simulink model "equation"  (R2020b)
settings: Solver=VariableStepAuto  StartTime=0.0  StopTime=10.0  RelTol=1e-3
settings Model: Creator=99003736  LastModifiedBy=99003736

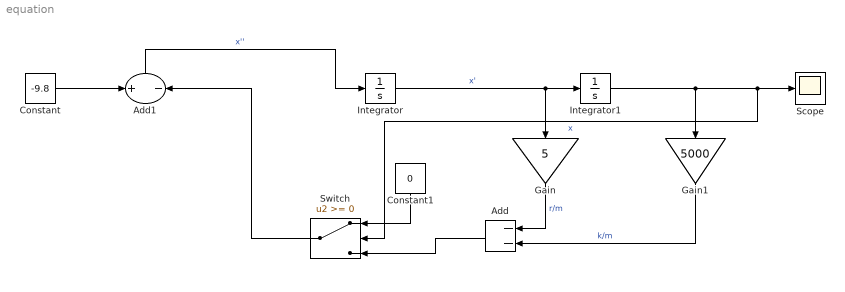
== system equation ==
  Add : Sum  Inputs=--
  Add1 : Sum  Inputs=+-
  Constant : Constant  Value=-9.8
  Constant1 : Constant  Value=0
  Gain : Gain  Gain=5
  Gain1 : Gain  Gain=5000
  Integrator : Integrator
  Integrator1 : Integrator
  Scope : Scope
  Switch : Switch
  wires:
  Integrator/1 -> Integrator1/1, Gain/1  "x'"
  Integrator1/1 -> Switch/2, Scope/1, Gain1/1  "x"
  Gain/1 -> Add/1  "r/m"
  Gain1/1 -> Add/2  "k/m"
  Switch/1 -> Add1/2
  Constant/1 -> Add1/1
  Add1/1 -> Integrator/1  "x''"
  Add/1 -> Switch/3
  Constant1/1 -> Switch/1
